simulink model "ASW_AST"  (R2023a)
settings: configuration reference "cfg_FastTaskCodeGeneration_v01" (kept outside this file)
undefined symbols (not defined in the file): Cdbl_tiSlwTaskSmpTi, Gu16_psiPermMagFlx_C
libraries: lib_conversion x1
settings Model: DataDictionary=dd_foc_dictionary.sldd  EnableAccessToBaseWorkspace=off  Creator=WFYXQ  LastModifiedBy=xiaoqiang.yuan
settings ConfigSetRef: SourceName=cfg_FastTaskCodeGeneration_v01

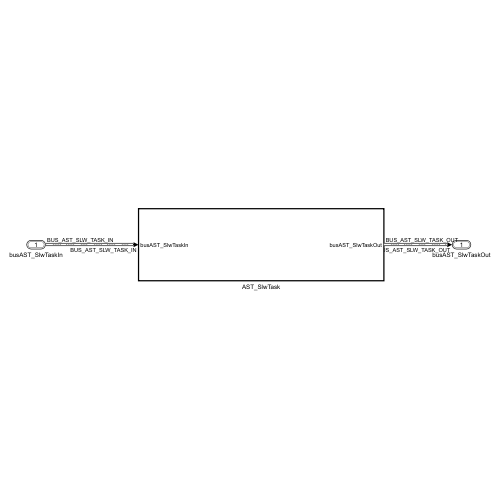
[thumbnail: Simulink's stored preview of the top-level diagram]
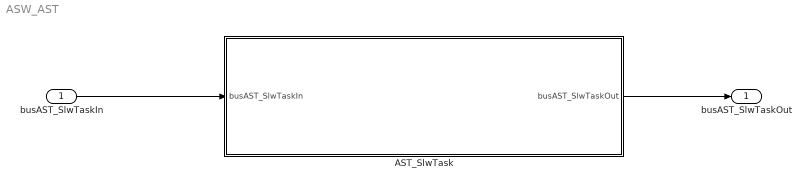
== system ASW_AST ==
  busAST_SlwTaskIn : Inport  OutDataTypeStr=Bus: BUS_AST_SLW_TASK_IN  SampleTime=round(double(Cdbl_tiSlwTaskSmpTi),4)  BusOutputAsStruct=on
  AST_SlwTask : Subsystem  TreatAsAtomicUnit=on  RTWFcnName=AST_SlwTask
      settings: RTWSystemCode=Nonreusable function  RTWFcnNameOpts=User specified
  busAST_SlwTaskOut : Outport  OutDataTypeStr=Bus: BUS_AST_SLW_TASK_OUT  SampleTime=round(double(Cdbl_tiSlwTaskSmpTi),4)
  wires:
  busAST_SlwTaskIn/1 -> AST_SlwTask/1(busAST_SlwTaskIn)
  AST_SlwTask/1(busAST_SlwTaskOut) -> busAST_SlwTaskOut/1

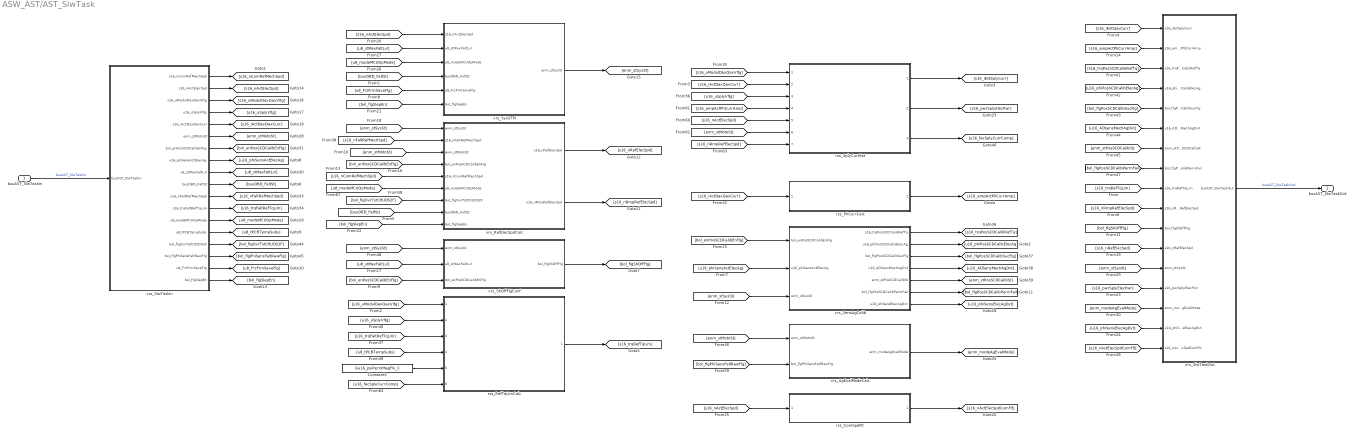
== system ASW_AST/AST_SlwTask ==
  busAST_SlwTaskIn : Inport
  Constant3 : Constant  Value=Gu16_psiPermMagFlx_C
  rss_ComSpdFlt : Subsystem  ReferencedSubsystem=rss_ComSpdFlt
  rss_PhCurrCalc : Subsystem  ReferencedSubsystem=rss_PhCurrCalc
  rss_RefTqLimCalc : Subsystem  ReferencedSubsystem=rss_RefTqLimCalc
  rss_SplyCurrEst : Subsystem  ReferencedSubsystem=rss_SplyCurrEst
  vrs_AgEvalModeCalc : Subsystem  Variant=on  VariantControlMode=label  VariantControl=Choice  LabelModeActiveChoice=cstHybrCtrlLbl
  vrs_RefElecSpdCalc : Subsystem  Variant=on  VariantControlMode=label  VariantControl=Choice  LabelModeActiveChoice=cstHybrCtrlLbl
  vrs_SensAgCalib : Subsystem  Variant=on  VariantControlMode=label  VariantControl=Choice  LabelModeActiveChoice=cstSensCtrlLbl
  vrs_ShOffFlgConf : Subsystem  Variant=on  VariantControlMode=label  VariantControl=Choice  LabelModeActiveChoice=cstSensCtrlLbl
  vrs_SlwTaskIn : Subsystem  Variant=on  VariantControlMode=label  VariantControl=cstSenlCtrlLbl  LabelModeActiveChoice=cstHybrCtrlLbl
  vrs_SlwTaskOut : Subsystem  Variant=on  VariantControlMode=label  VariantControl=Choice  LabelModeActiveChoice=cstHybrCtrlLbl
  vrs_SysSTM : Subsystem  Variant=on  VariantControlMode=label  VariantControl=Choice  LabelModeActiveChoice=GEELY_PROJECT
  busAST_SlwTaskOut : Outport
  wires:
  vrs_SensAgCalib/6(bol_flgPosSCDCalibPermFail) -> [bol_flgPosSCDCalibPermFail]
  vrs_SensAgCalib/5(enm_stPosSCDCalibSt) -> [enm_stPosSCDCalibSt]
  vrs_SensAgCalib/4(u16_ADSensMechAgDvt) -> [u16_ADSensMechAgDvt]
  vrs_SensAgCalib/2(u16_phiPosSCDCalibElecAg) -> [u16_phiPosSCDCalibElecAg]
  vrs_SensAgCalib/3(bol_flgPosSCDCalibSucFlg) -> [bol_flgPosSCDCalibSucFlg]
  [s16_iActDaxQaxCurr] -> rss_PhCurrCalc/1
  vrs_SlwTaskOut/1(busAST_SlwTaskOut) -> busAST_SlwTaskOut/1  "busAST_SlwTaskOut"
  [s16_iEstSplyCurr] -> vrs_SlwTaskOut/1(s16_iEstSplyCurr)
  [u16_uSplyVltg] -> rss_RefTqLimCalc/2
  [s16_uModulDaxQaxVltg] -> rss_SplyCurrEst/1
  rss_RefTqLimCalc/1 -> [s16_trqRefTqLim]
  rss_PhCurrCalc/1 -> [s16_ampActPhCurrAmp]
  [u16_uSplyVltg] -> rss_SplyCurrEst/3
  [s16_ampActPhCurrAmp] -> vrs_SlwTaskOut/2(s16_ampActPhCurrAmp)
  [bol_enPosSCDCalibEnFlg] -> vrs_SensAgCalib/1(bol_enPosSCDCalibEnFlg)
  [s16_iActDaxQaxCurr] -> rss_SplyCurrEst/2
  [s16_uModulDaxQaxVltg] -> rss_RefTqLimCalc/1
  [u16_phiPosSCDCalibElecAg] -> vrs_SlwTaskOut/4(u16_phiPosSCDCalibElecAg)
  [bol_flgPosSCDCalibPermFail] -> vrs_SlwTaskOut/8(bol_flgPosSCDCalibPermFail)
  [enm_stPosSCDCalibSt] -> vrs_SlwTaskOut/7(enm_stPosSCDCalibSt)
  [u16_ADSensMechAgDvt] -> vrs_SlwTaskOut/6(u16_ADSensMechAgDvt)
  [bol_flgPosSCDCalibSucFlg] -> vrs_SlwTaskOut/5(bol_flgPosSCDCalibSucFlg)
  [s16_trqPosSCDCalibRefTq] -> vrs_SlwTaskOut/3(s16_trqPosSCDCalibRefTq)
  vrs_SensAgCalib/1(s16_trqPosSCDCalibRefTq) -> [s16_trqPosSCDCalibRefTq]
  rss_SplyCurrEst/1 -> [s16_iEstSplyCurr]
  [s16_trqRefTqLim] -> vrs_SlwTaskOut/9(s16_trqRefTqLim)
  [s16_nRmpRefElecSpd] -> vrs_SlwTaskOut/10(s16_nRmpRefElecSpd)
  [bol_flgShOffFlg] -> vrs_SlwTaskOut/11(bol_flgShOffFlg)
  [u16_phiSensActElecAg] -> vrs_SensAgCalib/2(u16_phiSensActElecAg)
  [s16_nRefElecSpd] -> vrs_SlwTaskOut/12(s16_nRefElecSpd)
  [enm_stSysSt] -> vrs_SlwTaskOut/13(enm_stSysSt)
  [s16_trqFaltRefTqLim] -> rss_RefTqLimCalc/3
  [u8_tPCBTempSubs] -> rss_RefTqLimCalc/4
  [enm_stSysSt] -> vrs_SensAgCalib/3(enm_stSysSt)
  Constant3/1 -> rss_RefTqLimCalc/5
  [enm_stSysSt] -> vrs_ShOffFlgConf/1(enm_stSysSt)
  [u8_stMaxFaltLvl] -> vrs_ShOffFlgConf/2(u8_stMaxFaltLvl)
  [bol_enPosSCDCalibEnFlg] -> vrs_ShOffFlgConf/3(bol_enPosSCDCalibEnFlg)
  vrs_ShOffFlgConf/1(bol_flgShOffFlg) -> [bol_flgShOffFlg]
  [enm_stSysSt] -> vrs_RefElecSpdCalc/1(enm_stSysSt)
  [s16_nFaltRefMechSpd] -> vrs_RefElecSpdCalc/2(s16_nFaltRefMechSpd)
  [enm_stMotoSt] -> vrs_RefElecSpdCalc/3(enm_stMotoSt)
  [bol_enPosSCDCalibEnFlg] -> vrs_RefElecSpdCalc/4(bol_enPosSCDCalibEnFlg)
  [s16_nComRefMechSpd] -> vrs_RefElecSpdCalc/5(s16_nComRefMechSpd)
  vrs_RefElecSpdCalc/1(s16_nRefElecSpd) -> [s16_nRefElecSpd]
  vrs_RefElecSpdCalc/2(s16_nRmpRefElecSpd) -> [s16_nRmpRefElecSpd]
  [u8_modeMCUOpMode] -> vrs_RefElecSpdCalc/6(u8_modeMCUOpMode)
  rss_SplyCurrEst/2 -> [s16_pwrSplyElecPwr]
  [s16_pwrSplyElecPwr] -> vrs_SlwTaskOut/14(s16_pwrSplyElecPwr)
  [bol_flgOvrTstCtlUDS2F] -> vrs_RefElecSpdCalc/7(bol_flgOvrTstCtlUDS2F)
  [enm_modeAgEvalMode] -> vrs_SlwTaskOut/15(enm_modeAgEvalMode)
  busAST_SlwTaskIn/1 -> vrs_SlwTaskIn/1(busAST_SlwTaskIn)  "busAST_SlwTaskIn"
  vrs_SlwTaskIn/1(s16_nComRefMechSpd) -> [s16_nComRefMechSpd]
  vrs_SlwTaskIn/2(s16_nActElecSpd) -> [s16_nActElecSpd]
  vrs_SlwTaskIn/3(s16_uModulDaxQaxVltg) -> [s16_uModulDaxQaxVltg]
  vrs_SlwTaskIn/4(u16_uSplyVltg) -> [u16_uSplyVltg]
  vrs_SlwTaskIn/5(s16_iActDaxQaxCurr) -> [s16_iActDaxQaxCurr]
  vrs_SlwTaskIn/6(enm_stMotoSt) -> [enm_stMotoSt]
  vrs_SlwTaskIn/7(bol_enPosSCDCalibEnFlg) -> [bol_enPosSCDCalibEnFlg]
  vrs_SlwTaskIn/8(u16_phiSensActElecAg) -> [u16_phiSensActElecAg]
  vrs_SlwTaskIn/9(u8_stMaxFaltLvl) -> [u8_stMaxFaltLvl]
  vrs_SlwTaskIn/10(busOBD_FaltSt) -> [busOBD_FaltSt]
  vrs_SlwTaskIn/11(s16_nFaltRefMechSpd) -> [s16_nFaltRefMechSpd]
  vrs_SlwTaskIn/12(s16_trqFaltRefTqLim) -> [s16_trqFaltRefTqLim]
  vrs_SlwTaskIn/13(u8_modeMCUOpMode) -> [u8_modeMCUOpMode]
  vrs_SlwTaskIn/14(u8_tPCBTempSubs) -> [u8_tPCBTempSubs]
  vrs_SlwTaskIn/15(bol_flgOvrTstCtlUDS2F) -> [bol_flgOvrTstCtlUDS2F]
  vrs_AgEvalModeCalc/1(enm_modeAgEvalMode) -> [enm_modeAgEvalMode]
  [enm_stMotoSt] -> vrs_AgEvalModeCalc/1(enm_stMotoSt)
  [bol_flgPhiSensFaltRawFlg] -> vrs_AgEvalModeCalc/2(bol_flgPhiSensFaltRawFlg)
  vrs_SlwTaskIn/16(bol_flgPhiSensFaltRawFlg) -> [bol_flgPhiSensFaltRawFlg]
  [s16_ampActPhCurrAmp] -> rss_SplyCurrEst/4
  [s16_nActElecSpd] -> rss_SplyCurrEst/5
  [enm_stMotoSt] -> rss_SplyCurrEst/6
  [s16_nRmpRefElecSpd] -> rss_SplyCurrEst/7
  rss_SplyCurrEst/3 -> [u16_facSplyCurrComp]
  [u16_facSplyCurrComp] -> rss_RefTqLimCalc/6
  [busOBD_FaltSt] -> vrs_RefElecSpdCalc/8(busOBD_FaltSt)
  vrs_SlwTaskIn/17(u8_FrzFrmSaveFlg) -> [u8_FrzFrmSaveFlg]
  [s16_nActElecSpd] -> vrs_SysSTM/1(s16_nActElecSpd)
  [u8_stMaxFaltLvl] -> vrs_SysSTM/2(u8_stMaxFaltLvl)
  [u8_modeMCUOpMode] -> vrs_SysSTM/3(u8_modeMCUOpMode)
  [busOBD_FaltSt] -> vrs_SysSTM/4(busOBD_FaltSt)
  [u8_FrzFrmSaveFlg] -> vrs_SysSTM/5(u8_FrzFrmSaveFlg)
  vrs_SysSTM/1(enm_stSysSt) -> [enm_stSysSt]
  [bol_flgSlepEn] -> vrs_SysSTM/6(bol_flgSlepEn)
  [bol_flgSlepEn] -> vrs_RefElecSpdCalc/9(bol_flgSlepEn)
  vrs_SlwTaskIn/18(bol_flgSlepEn) -> [bol_flgSlepEn]
  vrs_SensAgCalib/7(u16_phiSensElecAgDvt) -> [u16_phiSensElecAgDvt]
  [u16_phiSensElecAgDvt] -> vrs_SlwTaskOut/16(u16_phiSensElecAgDvt)
  [s16_nActElecSpd] -> rss_ComSpdFlt/1
  rss_ComSpdFlt/1 -> [s16_nActElecSpdComFlt]
  [s16_nActElecSpdComFlt] -> vrs_SlwTaskOut/17(s16_nActElecSpdComFlt)

== system ASW_AST/AST_SlwTask/vrs_AgEvalModeCalc ==
  enm_stMotoSt : Inport
  bol_flgPhiSensFaltRawFlg : Inport  Port=2
  rss_AgEvalModeCalcNeed : Subsystem  VariantControl=cstHybrCtrlLbl  ReferencedSubsystem=rss_AgEvalModeCalcNeed
  rss_AgEvalModeCalcNoNeed : Subsystem  VariantControl=cstSensCtrlLbl
  enm_modeAgEvalMode : Outport

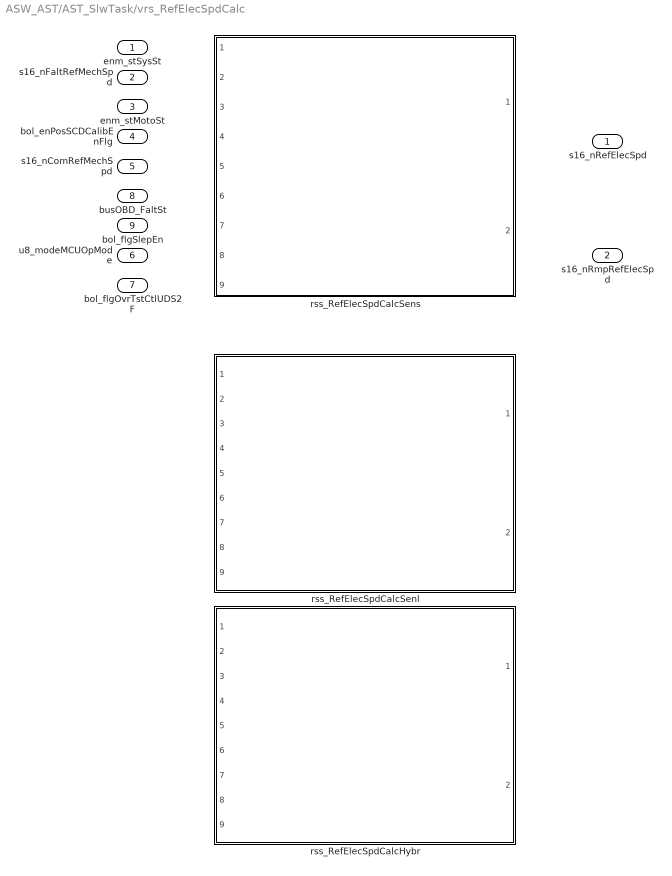
== system ASW_AST/AST_SlwTask/vrs_RefElecSpdCalc ==
  enm_stSysSt : Inport
  s16_nFaltRefMechSpd : Inport  Port=2
  enm_stMotoSt : Inport  Port=3
  bol_enPosSCDCalibEnFlg : Inport  Port=4
  s16_nComRefMechSpd : Inport  Port=5
  u8_modeMCUOpMode : Inport  Port=6
  bol_flgOvrTstCtlUDS2F : Inport  Port=7  OutDataTypeStr=boolean
  busOBD_FaltSt : Inport  Port=8  OutDataTypeStr=Bus: BUS_OBD_FALT_STS
  bol_flgSlepEn : Inport  Port=9
  rss_RefElecSpdCalcHybr : Subsystem  VariantControl=cstHybrCtrlLbl  ReferencedSubsystem=rss_RefElecSpdCalcHybr
  rss_RefElecSpdCalcSenl : Subsystem  VariantControl=cstSenlCtrlLbl  ReferencedSubsystem=rss_RefElecSpdCalcSenl
  rss_RefElecSpdCalcSens : Subsystem  VariantControl=cstSensCtrlLbl  ReferencedSubsystem=rss_RefElecSpdCalcSens
  s16_nRefElecSpd : Outport
  s16_nRmpRefElecSpd : Outport  Port=2

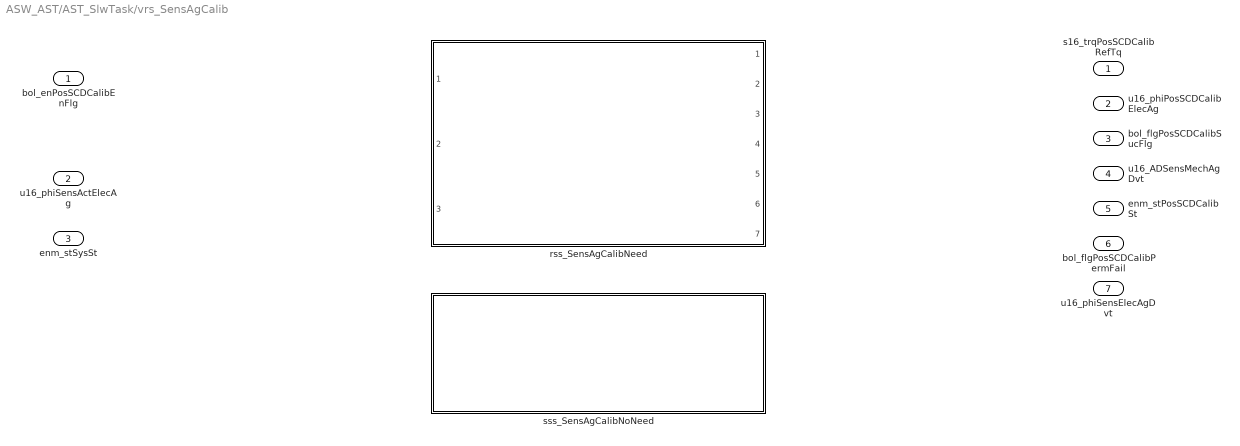
== system ASW_AST/AST_SlwTask/vrs_SensAgCalib ==
  bol_enPosSCDCalibEnFlg : Inport
  u16_phiSensActElecAg : Inport  Port=2
  enm_stSysSt : Inport  Port=3
  rss_SensAgCalibNeed : Subsystem  VariantControl=cstSensCtrlLbl  ReferencedSubsystem=rss_SensAgCalibNeed
  sss_SensAgCalibNoNeed : Subsystem  VariantControl=cstSenlCtrlLbl
  s16_trqPosSCDCalibRefTq : Outport
  u16_phiPosSCDCalibElecAg : Outport  Port=2
  bol_flgPosSCDCalibSucFlg : Outport  Port=3
  u16_ADSensMechAgDvt : Outport  Port=4
  enm_stPosSCDCalibSt : Outport  Port=5
  bol_flgPosSCDCalibPermFail : Outport  Port=6
  u16_phiSensElecAgDvt : Outport  Port=7

== system ASW_AST/AST_SlwTask/vrs_ShOffFlgConf ==
  enm_stSysSt : Inport
  u8_stMaxFaltLvl : Inport  Port=2
  bol_enPosSCDCalibEnFlg : Inport  Port=3
  rss_ShOffFlgConfSenl : Subsystem  VariantControl=cstSenlCtrlLbl  ReferencedSubsystem=rss_ShOffFlgConfSenl
  rss_ShOffFlgConfSens : Subsystem  VariantControl=cstSensCtrlLbl  ReferencedSubsystem=rss_ShOffFlgConfSens
  bol_flgShOffFlg : Outport

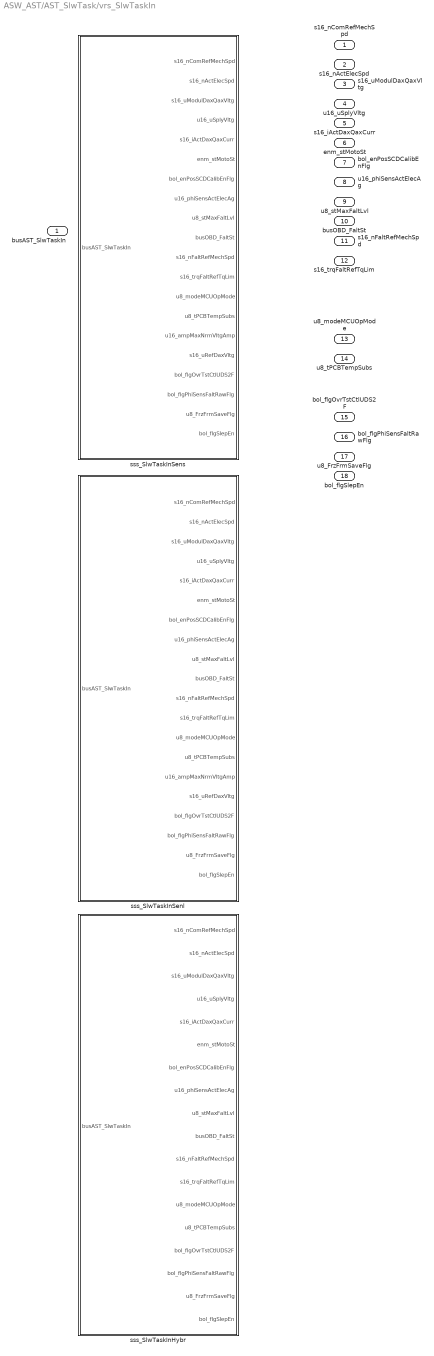
== system ASW_AST/AST_SlwTask/vrs_SlwTaskIn ==
  busAST_SlwTaskIn : Inport
  sss_SlwTaskInHybr : Subsystem  VariantControl=cstHybrCtrlLbl
  sss_SlwTaskInSenl : Subsystem  VariantControl=cstSenlCtrlLbl
  sss_SlwTaskInSens : Subsystem  VariantControl=cstSensCtrlLbl
  s16_nComRefMechSpd : Outport
  s16_nActElecSpd : Outport  Port=2
  s16_uModulDaxQaxVltg : Outport  Port=3
  u16_uSplyVltg : Outport  Port=4
  s16_iActDaxQaxCurr : Outport  Port=5
  enm_stMotoSt : Outport  Port=6
  bol_enPosSCDCalibEnFlg : Outport  Port=7
  u16_phiSensActElecAg : Outport  Port=8
  u8_stMaxFaltLvl : Outport  Port=9
  busOBD_FaltSt : Outport  Port=10
  s16_nFaltRefMechSpd : Outport  Port=11
  s16_trqFaltRefTqLim : Outport  Port=12
  u8_modeMCUOpMode : Outport  Port=13
  u8_tPCBTempSubs : Outport  Port=14
  bol_flgOvrTstCtlUDS2F : Outport  Port=15
  bol_flgPhiSensFaltRawFlg : Outport  Port=16
  u8_FrzFrmSaveFlg : Outport  Port=17
  bol_flgSlepEn : Outport  Port=18

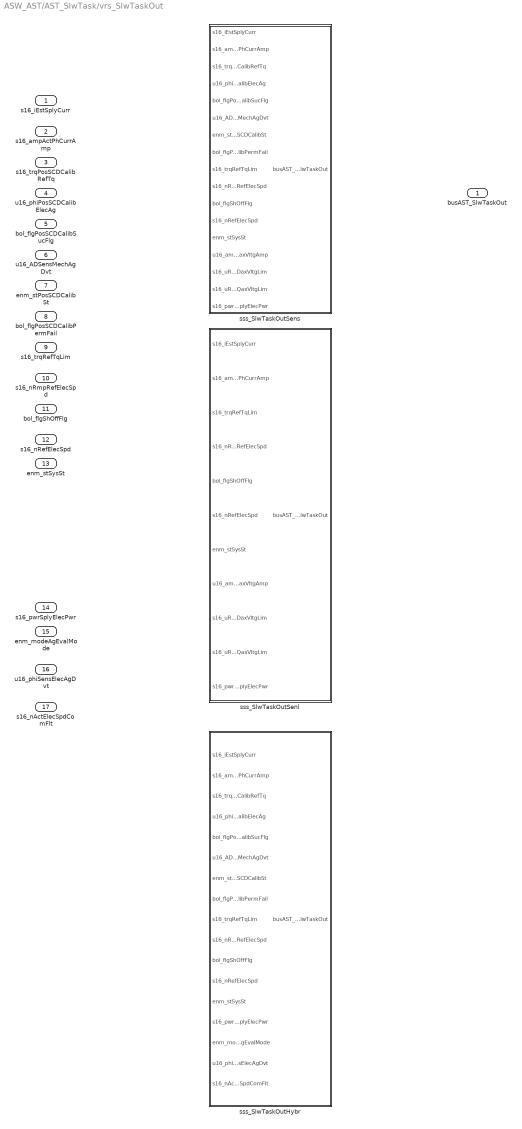
== system ASW_AST/AST_SlwTask/vrs_SlwTaskOut ==
  s16_iEstSplyCurr : Inport
  s16_ampActPhCurrAmp : Inport  Port=2
  s16_trqPosSCDCalibRefTq : Inport  Port=3
  u16_phiPosSCDCalibElecAg : Inport  Port=4
  bol_flgPosSCDCalibSucFlg : Inport  Port=5
  u16_ADSensMechAgDvt : Inport  Port=6
  enm_stPosSCDCalibSt : Inport  Port=7
  bol_flgPosSCDCalibPermFail : Inport  Port=8
  s16_trqRefTqLim : Inport  Port=9
  s16_nRmpRefElecSpd : Inport  Port=10
  bol_flgShOffFlg : Inport  Port=11
  s16_nRefElecSpd : Inport  Port=12
  enm_stSysSt : Inport  Port=13
  s16_pwrSplyElecPwr : Inport  Port=14
  enm_modeAgEvalMode : Inport  Port=15
  u16_phiSensElecAgDvt : Inport  Port=16
  s16_nActElecSpdComFlt : Inport  Port=17
  sss_SlwTaskOutHybr : Subsystem  VariantControl=cstHybrCtrlLbl
  sss_SlwTaskOutSenl : Subsystem  VariantControl=cstSenlCtrlLbl
  sss_SlwTaskOutSens : Subsystem  VariantControl=cstSensCtrlLbl
  busAST_SlwTaskOut : Outport

== system ASW_AST/AST_SlwTask/vrs_SysSTM ==
  s16_nActElecSpd : Inport
  u8_stMaxFaltLvl : Inport  Port=2
  u8_modeMCUOpMode : Inport  Port=3
  busOBD_FaltSt : Inport  Port=4
  u8_FrzFrmSaveFlg : Inport  Port=5
  bol_flgSlepEn : Inport  Port=6
  rss_SysSTM_CRRC : Subsystem  VariantControl=CRRC_PROJECT  ReferencedSubsystem=rss_SysSTM_CRRC
  rss_SysSTM_GEELY : Subsystem  VariantControl=GEELY_PROJECT  ReferencedSubsystem=rss_SysSTM_GEELY
  enm_stSysSt : Outport

== system ASW_AST/AST_SlwTask/vrs_AgEvalModeCalc/rss_AgEvalModeCalcNoNeed ==
  enm_stMotoSt : Inport  OutDataTypeStr=Enum: ENM_MOTO_STATUS
  bol_flgPhiSensFaltRawFlg : Inport  Port=2  OutDataTypeStr=boolean
  Ground : Ground
  Terminator : Terminator
  Terminator1 : Terminator
  lib_Cnvr_3 : lib_conversion/lib_Conversion_0  lb_parDataType=Inherit: Inherit via back propagation  lb_parOutpMaxVal=[]  lb_parOutpMinVal=[]  lb_parSatFlag=off
  enm_modeAgEvalMode : Outport
  wires:
  enm_stMotoSt/1 -> Terminator/1
  bol_flgPhiSensFaltRawFlg/1 -> Terminator1/1
  Ground/1 -> lib_Cnvr_3/1
  lib_Cnvr_3/1 -> enm_modeAgEvalMode/1

== system ASW_AST/AST_SlwTask/vrs_SensAgCalib/sss_SensAgCalibNoNeed ==

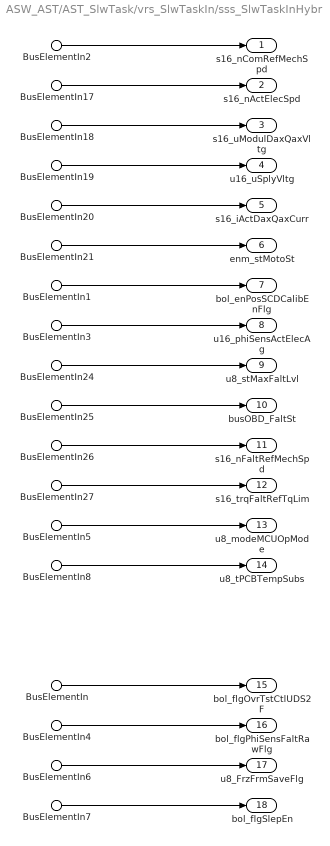
== system ASW_AST/AST_SlwTask/vrs_SlwTaskIn/sss_SlwTaskInHybr ==
  BusElementIn2 : Inport  PortName=busAST_SlwTaskIn  Element=s16_nComRefMechSpd
  BusElementIn17 : Inport  PortName=busAST_SlwTaskIn  Element=s16_nActElecSpd
  BusElementIn18 : Inport  PortName=busAST_SlwTaskIn  Element=s16_uModulDaxQaxVltg
  BusElementIn19 : Inport  PortName=busAST_SlwTaskIn  Element=u16_uSplyVltg
  BusElementIn20 : Inport  PortName=busAST_SlwTaskIn  Element=s16_iActDaxQaxCurr
  BusElementIn21 : Inport  PortName=busAST_SlwTaskIn  Element=enm_stMotoSt
  BusElementIn24 : Inport  PortName=busAST_SlwTaskIn  Element=u8_stMaxFaltLvl
  BusElementIn25 : Inport  PortName=busAST_SlwTaskIn  Element=busOBD_FaltSt
  BusElementIn26 : Inport  PortName=busAST_SlwTaskIn  Element=s16_nFaltRefMechSpd
  BusElementIn27 : Inport  PortName=busAST_SlwTaskIn  Element=s16_trqFaltRefTqLim
  BusElementIn : Inport  PortName=busAST_SlwTaskIn  Element=bol_flgOvrTstCtlUDS2F
  BusElementIn1 : Inport  PortName=busAST_SlwTaskIn  Element=bol_enPosSCDCalibEnFlg
  BusElementIn3 : Inport  PortName=busAST_SlwTaskIn  Element=u16_phiSensActElecAg
  BusElementIn4 : Inport  PortName=busAST_SlwTaskIn  Element=bol_flgPhiSensFaltRawFlg
  BusElementIn5 : Inport  PortName=busAST_SlwTaskIn  Element=u8_modeMCUOpMode
  BusElementIn6 : Inport  PortName=busAST_SlwTaskIn  Element=u8_FrzFrmSaveFlg
  BusElementIn7 : Inport  PortName=busAST_SlwTaskIn  Element=bol_flgSlepEn
  BusElementIn8 : Inport  PortName=busAST_SlwTaskIn  Element=u8_tPCBTempSubs
  s16_nComRefMechSpd : Outport
  s16_nActElecSpd : Outport  Port=2
  s16_uModulDaxQaxVltg : Outport  Port=3
  u16_uSplyVltg : Outport  Port=4
  s16_iActDaxQaxCurr : Outport  Port=5
  enm_stMotoSt : Outport  Port=6
  bol_enPosSCDCalibEnFlg : Outport  Port=7
  u16_phiSensActElecAg : Outport  Port=8
  u8_stMaxFaltLvl : Outport  Port=9
  busOBD_FaltSt : Outport  Port=10
  s16_nFaltRefMechSpd : Outport  Port=11
  s16_trqFaltRefTqLim : Outport  Port=12
  u8_modeMCUOpMode : Outport  Port=13
  u8_tPCBTempSubs : Outport  Port=14
  bol_flgOvrTstCtlUDS2F : Outport  Port=15
  bol_flgPhiSensFaltRawFlg : Outport  Port=16
  u8_FrzFrmSaveFlg : Outport  Port=17
  bol_flgSlepEn : Outport  Port=18
  wires:
  BusElementIn/1 -> bol_flgOvrTstCtlUDS2F/1
  BusElementIn21/1 -> enm_stMotoSt/1
  BusElementIn24/1 -> u8_stMaxFaltLvl/1
  BusElementIn25/1 -> busOBD_FaltSt/1
  BusElementIn26/1 -> s16_nFaltRefMechSpd/1
  BusElementIn27/1 -> s16_trqFaltRefTqLim/1
  BusElementIn5/1 -> u8_modeMCUOpMode/1
  BusElementIn8/1 -> u8_tPCBTempSubs/1
  BusElementIn20/1 -> s16_iActDaxQaxCurr/1
  BusElementIn19/1 -> u16_uSplyVltg/1
  BusElementIn18/1 -> s16_uModulDaxQaxVltg/1
  BusElementIn17/1 -> s16_nActElecSpd/1
  BusElementIn2/1 -> s16_nComRefMechSpd/1
  BusElementIn1/1 -> bol_enPosSCDCalibEnFlg/1
  BusElementIn3/1 -> u16_phiSensActElecAg/1
  BusElementIn4/1 -> bol_flgPhiSensFaltRawFlg/1
  BusElementIn6/1 -> u8_FrzFrmSaveFlg/1
  BusElementIn7/1 -> bol_flgSlepEn/1

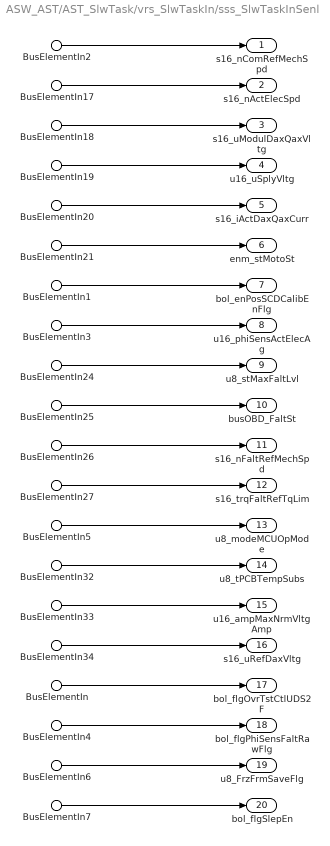
== system ASW_AST/AST_SlwTask/vrs_SlwTaskIn/sss_SlwTaskInSenl ==
  BusElementIn2 : Inport  PortName=busAST_SlwTaskIn  Element=s16_nComRefMechSpd
  BusElementIn17 : Inport  PortName=busAST_SlwTaskIn  Element=s16_nActElecSpd
  BusElementIn18 : Inport  PortName=busAST_SlwTaskIn  Element=s16_uModulDaxQaxVltg
  BusElementIn19 : Inport  PortName=busAST_SlwTaskIn  Element=u16_uSplyVltg
  BusElementIn20 : Inport  PortName=busAST_SlwTaskIn  Element=s16_iActDaxQaxCurr
  BusElementIn21 : Inport  PortName=busAST_SlwTaskIn  Element=enm_stMotoSt
  BusElementIn24 : Inport  PortName=busAST_SlwTaskIn  Element=u8_stMaxFaltLvl
  BusElementIn25 : Inport  PortName=busAST_SlwTaskIn  Element=busOBD_FaltSt
  BusElementIn26 : Inport  PortName=busAST_SlwTaskIn  Element=s16_nFaltRefMechSpd
  BusElementIn27 : Inport  PortName=busAST_SlwTaskIn  Element=s16_trqFaltRefTqLim
  BusElementIn32 : Inport  PortName=busAST_SlwTaskIn  Element=u8_tPCBTemp
  BusElementIn33 : Inport  PortName=busAST_SlwTaskIn  Element=u16_ampMaxNrmVltgAmp
  BusElementIn34 : Inport  PortName=busAST_SlwTaskIn  Element=s16_uRefDaxVltg
  BusElementIn : Inport  PortName=busAST_SlwTaskIn  Element=bol_flgOvrTstCtlUDS2F
  BusElementIn1 : Inport  PortName=busAST_SlwTaskIn  Element=bol_enPosSCDCalibEnFlg
  BusElementIn3 : Inport  PortName=busAST_SlwTaskIn  Element=u16_phiSensActElecAg
  BusElementIn4 : Inport  PortName=busAST_SlwTaskIn  Element=bol_flgPhiSensFaltRawFlg
  BusElementIn5 : Inport  PortName=busAST_SlwTaskIn  Element=u8_modeMCUOpMode
  BusElementIn6 : Inport  PortName=busAST_SlwTaskIn  Element=u8_FrzFrmSaveFlg
  BusElementIn7 : Inport  PortName=busAST_SlwTaskIn  Element=bol_flgSlepEn
  s16_nComRefMechSpd : Outport
  s16_nActElecSpd : Outport  Port=2
  s16_uModulDaxQaxVltg : Outport  Port=3
  u16_uSplyVltg : Outport  Port=4
  s16_iActDaxQaxCurr : Outport  Port=5
  enm_stMotoSt : Outport  Port=6
  bol_enPosSCDCalibEnFlg : Outport  Port=7
  u16_phiSensActElecAg : Outport  Port=8
  u8_stMaxFaltLvl : Outport  Port=9
  busOBD_FaltSt : Outport  Port=10
  s16_nFaltRefMechSpd : Outport  Port=11
  s16_trqFaltRefTqLim : Outport  Port=12
  u8_modeMCUOpMode : Outport  Port=13
  u8_tPCBTempSubs : Outport  Port=14
  u16_ampMaxNrmVltgAmp : Outport  Port=15
  s16_uRefDaxVltg : Outport  Port=16
  bol_flgOvrTstCtlUDS2F : Outport  Port=17
  bol_flgPhiSensFaltRawFlg : Outport  Port=18
  u8_FrzFrmSaveFlg : Outport  Port=19
  bol_flgSlepEn : Outport  Port=20
  wires:
  BusElementIn17/1 -> s16_nActElecSpd/1
  BusElementIn7/1 -> bol_flgSlepEn/1
  BusElementIn2/1 -> s16_nComRefMechSpd/1
  BusElementIn18/1 -> s16_uModulDaxQaxVltg/1
  BusElementIn3/1 -> u16_phiSensActElecAg/1
  BusElementIn1/1 -> bol_enPosSCDCalibEnFlg/1
  BusElementIn6/1 -> u8_FrzFrmSaveFlg/1
  BusElementIn/1 -> bol_flgOvrTstCtlUDS2F/1
  BusElementIn34/1 -> s16_uRefDaxVltg/1
  BusElementIn4/1 -> bol_flgPhiSensFaltRawFlg/1
  BusElementIn20/1 -> s16_iActDaxQaxCurr/1
  BusElementIn19/1 -> u16_uSplyVltg/1
  BusElementIn24/1 -> u8_stMaxFaltLvl/1
  BusElementIn32/1 -> u8_tPCBTempSubs/1
  BusElementIn27/1 -> s16_trqFaltRefTqLim/1
  BusElementIn25/1 -> busOBD_FaltSt/1
  BusElementIn26/1 -> s16_nFaltRefMechSpd/1
  BusElementIn21/1 -> enm_stMotoSt/1
  BusElementIn5/1 -> u8_modeMCUOpMode/1
  BusElementIn33/1 -> u16_ampMaxNrmVltgAmp/1

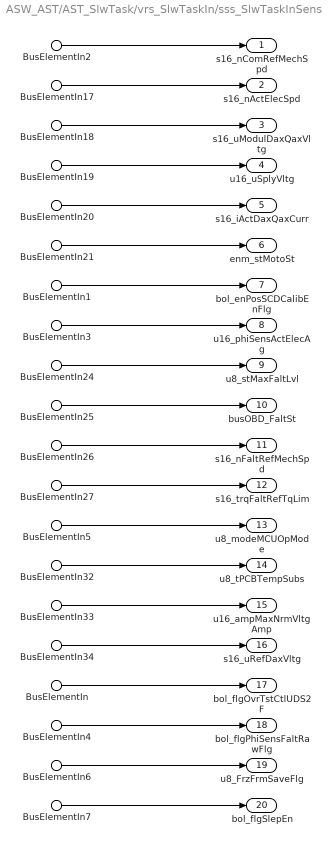
== system ASW_AST/AST_SlwTask/vrs_SlwTaskIn/sss_SlwTaskInSens ==
  BusElementIn2 : Inport  PortName=busAST_SlwTaskIn  Element=s16_nComRefMechSpd
  BusElementIn17 : Inport  PortName=busAST_SlwTaskIn  Element=s16_nActElecSpd
  BusElementIn18 : Inport  PortName=busAST_SlwTaskIn  Element=s16_uModulDaxQaxVltg
  BusElementIn19 : Inport  PortName=busAST_SlwTaskIn  Element=u16_uSplyVltg
  BusElementIn20 : Inport  PortName=busAST_SlwTaskIn  Element=s16_iActDaxQaxCurr
  BusElementIn21 : Inport  PortName=busAST_SlwTaskIn  Element=enm_stMotoSt
  BusElementIn24 : Inport  PortName=busAST_SlwTaskIn  Element=u8_stMaxFaltLvl
  BusElementIn25 : Inport  PortName=busAST_SlwTaskIn  Element=busOBD_FaltSt
  BusElementIn26 : Inport  PortName=busAST_SlwTaskIn  Element=s16_nFaltRefMechSpd
  BusElementIn27 : Inport  PortName=busAST_SlwTaskIn  Element=s16_trqFaltRefTqLim
  BusElementIn32 : Inport  PortName=busAST_SlwTaskIn  Element=u8_tPCBTemp
  BusElementIn33 : Inport  PortName=busAST_SlwTaskIn  Element=u16_ampMaxNrmVltgAmp
  BusElementIn34 : Inport  PortName=busAST_SlwTaskIn  Element=s16_uRefDaxVltg
  BusElementIn : Inport  PortName=busAST_SlwTaskIn  Element=bol_flgOvrTstCtlUDS2F
  BusElementIn1 : Inport  PortName=busAST_SlwTaskIn  Element=bol_enPosSCDCalibEnFlg
  BusElementIn3 : Inport  PortName=busAST_SlwTaskIn  Element=u16_phiSensActElecAg
  BusElementIn4 : Inport  PortName=busAST_SlwTaskIn  Element=bol_flgPhiSensFaltRawFlg
  BusElementIn5 : Inport  PortName=busAST_SlwTaskIn  Element=u8_modeMCUOpMode
  BusElementIn6 : Inport  PortName=busAST_SlwTaskIn  Element=u8_FrzFrmSaveFlg
  BusElementIn7 : Inport  PortName=busAST_SlwTaskIn  Element=bol_flgSlepEn
  s16_nComRefMechSpd : Outport
  s16_nActElecSpd : Outport  Port=2
  s16_uModulDaxQaxVltg : Outport  Port=3
  u16_uSplyVltg : Outport  Port=4
  s16_iActDaxQaxCurr : Outport  Port=5
  enm_stMotoSt : Outport  Port=6
  bol_enPosSCDCalibEnFlg : Outport  Port=7
  u16_phiSensActElecAg : Outport  Port=8
  u8_stMaxFaltLvl : Outport  Port=9
  busOBD_FaltSt : Outport  Port=10
  s16_nFaltRefMechSpd : Outport  Port=11
  s16_trqFaltRefTqLim : Outport  Port=12
  u8_modeMCUOpMode : Outport  Port=13
  u8_tPCBTempSubs : Outport  Port=14
  u16_ampMaxNrmVltgAmp : Outport  Port=15
  s16_uRefDaxVltg : Outport  Port=16
  bol_flgOvrTstCtlUDS2F : Outport  Port=17
  bol_flgPhiSensFaltRawFlg : Outport  Port=18
  u8_FrzFrmSaveFlg : Outport  Port=19
  bol_flgSlepEn : Outport  Port=20
  wires:
  BusElementIn17/1 -> s16_nActElecSpd/1
  BusElementIn7/1 -> bol_flgSlepEn/1
  BusElementIn2/1 -> s16_nComRefMechSpd/1
  BusElementIn18/1 -> s16_uModulDaxQaxVltg/1
  BusElementIn3/1 -> u16_phiSensActElecAg/1
  BusElementIn1/1 -> bol_enPosSCDCalibEnFlg/1
  BusElementIn6/1 -> u8_FrzFrmSaveFlg/1
  BusElementIn/1 -> bol_flgOvrTstCtlUDS2F/1
  BusElementIn34/1 -> s16_uRefDaxVltg/1
  BusElementIn4/1 -> bol_flgPhiSensFaltRawFlg/1
  BusElementIn20/1 -> s16_iActDaxQaxCurr/1
  BusElementIn19/1 -> u16_uSplyVltg/1
  BusElementIn24/1 -> u8_stMaxFaltLvl/1
  BusElementIn32/1 -> u8_tPCBTempSubs/1
  BusElementIn27/1 -> s16_trqFaltRefTqLim/1
  BusElementIn25/1 -> busOBD_FaltSt/1
  BusElementIn26/1 -> s16_nFaltRefMechSpd/1
  BusElementIn21/1 -> enm_stMotoSt/1
  BusElementIn5/1 -> u8_modeMCUOpMode/1
  BusElementIn33/1 -> u16_ampMaxNrmVltgAmp/1

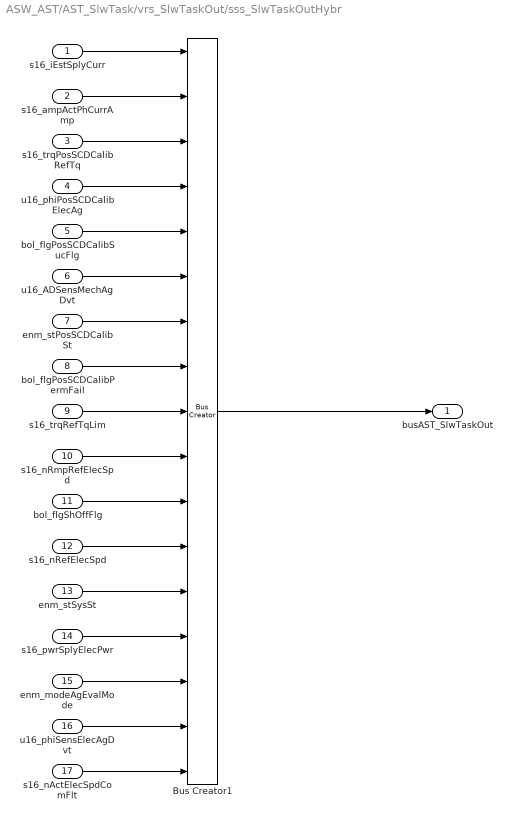
== system ASW_AST/AST_SlwTask/vrs_SlwTaskOut/sss_SlwTaskOutHybr ==
  s16_iEstSplyCurr : Inport
  s16_ampActPhCurrAmp : Inport  Port=2
  s16_trqPosSCDCalibRefTq : Inport  Port=3
  u16_phiPosSCDCalibElecAg : Inport  Port=4
  bol_flgPosSCDCalibSucFlg : Inport  Port=5
  u16_ADSensMechAgDvt : Inport  Port=6
  enm_stPosSCDCalibSt : Inport  Port=7
  bol_flgPosSCDCalibPermFail : Inport  Port=8
  s16_trqRefTqLim : Inport  Port=9
  s16_nRmpRefElecSpd : Inport  Port=10
  bol_flgShOffFlg : Inport  Port=11
  s16_nRefElecSpd : Inport  Port=12
  enm_stSysSt : Inport  Port=13
  s16_pwrSplyElecPwr : Inport  Port=14
  enm_modeAgEvalMode : Inport  Port=15
  u16_phiSensElecAgDvt : Inport  Port=16
  s16_nActElecSpdComFlt : Inport  Port=17
  Bus Creator1 : BusCreator  Inputs=17  OutDataTypeStr=Bus: BUS_AST_SLW_TASK_OUT  NonVirtualBus=on
      settings: InheritFromInputs=off
  busAST_SlwTaskOut : Outport
  wires:
  u16_phiPosSCDCalibElecAg/1 -> Bus Creator1/4
  bol_flgShOffFlg/1 -> Bus Creator1/11
  bol_flgPosSCDCalibSucFlg/1 -> Bus Creator1/5
  enm_stPosSCDCalibSt/1 -> Bus Creator1/7
  s16_ampActPhCurrAmp/1 -> Bus Creator1/2
  bol_flgPosSCDCalibPermFail/1 -> Bus Creator1/8
  s16_trqRefTqLim/1 -> Bus Creator1/9
  s16_trqPosSCDCalibRefTq/1 -> Bus Creator1/3
  s16_nRmpRefElecSpd/1 -> Bus Creator1/10
  Bus Creator1/1 -> busAST_SlwTaskOut/1
  u16_ADSensMechAgDvt/1 -> Bus Creator1/6
  s16_iEstSplyCurr/1 -> Bus Creator1/1
  s16_nRefElecSpd/1 -> Bus Creator1/12
  enm_stSysSt/1 -> Bus Creator1/13
  s16_pwrSplyElecPwr/1 -> Bus Creator1/14
  enm_modeAgEvalMode/1 -> Bus Creator1/15
  u16_phiSensElecAgDvt/1 -> Bus Creator1/16
  s16_nActElecSpdComFlt/1 -> Bus Creator1/17

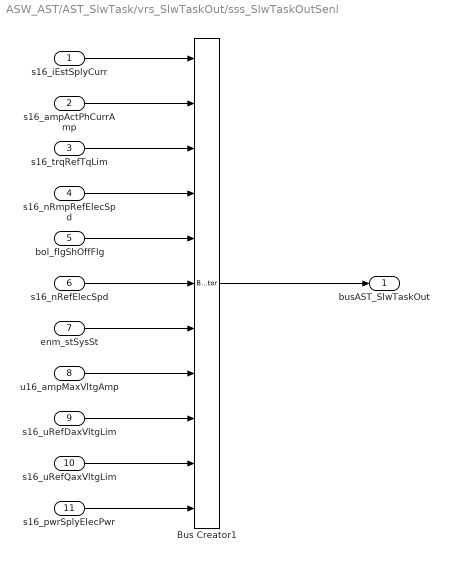
== system ASW_AST/AST_SlwTask/vrs_SlwTaskOut/sss_SlwTaskOutSenl ==
  s16_iEstSplyCurr : Inport
  s16_ampActPhCurrAmp : Inport  Port=2
  s16_trqRefTqLim : Inport  Port=3
  s16_nRmpRefElecSpd : Inport  Port=4
  bol_flgShOffFlg : Inport  Port=5
  s16_nRefElecSpd : Inport  Port=6
  enm_stSysSt : Inport  Port=7
  u16_ampMaxVltgAmp : Inport  Port=8
  s16_uRefDaxVltgLim : Inport  Port=9
  s16_uRefQaxVltgLim : Inport  Port=10
  s16_pwrSplyElecPwr : Inport  Port=11
  Bus Creator1 : BusCreator  Inputs=11  OutDataTypeStr=Bus: BUS_AST_SLW_TASK_OUT  NonVirtualBus=on
      settings: InheritFromInputs=off
  busAST_SlwTaskOut : Outport
  wires:
  Bus Creator1/1 -> busAST_SlwTaskOut/1
  s16_iEstSplyCurr/1 -> Bus Creator1/1
  s16_ampActPhCurrAmp/1 -> Bus Creator1/2
  s16_trqRefTqLim/1 -> Bus Creator1/3
  s16_nRmpRefElecSpd/1 -> Bus Creator1/4
  bol_flgShOffFlg/1 -> Bus Creator1/5
  s16_nRefElecSpd/1 -> Bus Creator1/6
  enm_stSysSt/1 -> Bus Creator1/7
  u16_ampMaxVltgAmp/1 -> Bus Creator1/8
  s16_uRefDaxVltgLim/1 -> Bus Creator1/9
  s16_uRefQaxVltgLim/1 -> Bus Creator1/10
  s16_pwrSplyElecPwr/1 -> Bus Creator1/11

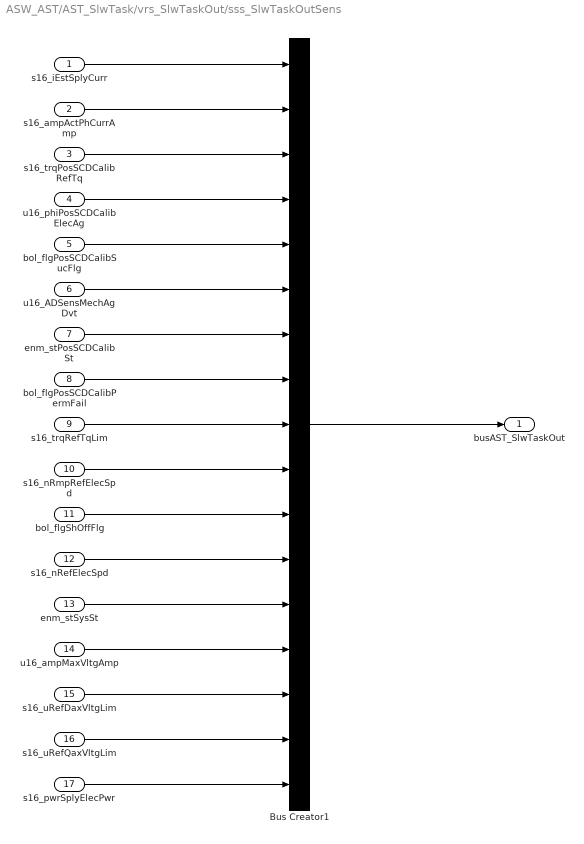
== system ASW_AST/AST_SlwTask/vrs_SlwTaskOut/sss_SlwTaskOutSens ==
  s16_iEstSplyCurr : Inport
  s16_ampActPhCurrAmp : Inport  Port=2
  s16_trqPosSCDCalibRefTq : Inport  Port=3
  u16_phiPosSCDCalibElecAg : Inport  Port=4
  bol_flgPosSCDCalibSucFlg : Inport  Port=5
  u16_ADSensMechAgDvt : Inport  Port=6
  enm_stPosSCDCalibSt : Inport  Port=7
  bol_flgPosSCDCalibPermFail : Inport  Port=8
  s16_trqRefTqLim : Inport  Port=9
  s16_nRmpRefElecSpd : Inport  Port=10
  bol_flgShOffFlg : Inport  Port=11
  s16_nRefElecSpd : Inport  Port=12
  enm_stSysSt : Inport  Port=13
  u16_ampMaxVltgAmp : Inport  Port=14
  s16_uRefDaxVltgLim : Inport  Port=15
  s16_uRefQaxVltgLim : Inport  Port=16
  s16_pwrSplyElecPwr : Inport  Port=17
  Bus Creator1 : BusCreator  Inputs=17  OutDataTypeStr=Bus: BUS_AST_SLW_TASK_OUT  NonVirtualBus=on
      settings: InheritFromInputs=off
  busAST_SlwTaskOut : Outport
  wires:
  s16_iEstSplyCurr/1 -> Bus Creator1/1
  s16_ampActPhCurrAmp/1 -> Bus Creator1/2
  s16_trqPosSCDCalibRefTq/1 -> Bus Creator1/3
  u16_phiPosSCDCalibElecAg/1 -> Bus Creator1/4
  bol_flgPosSCDCalibSucFlg/1 -> Bus Creator1/5
  u16_ADSensMechAgDvt/1 -> Bus Creator1/6
  enm_stPosSCDCalibSt/1 -> Bus Creator1/7
  bol_flgPosSCDCalibPermFail/1 -> Bus Creator1/8
  s16_trqRefTqLim/1 -> Bus Creator1/9
  s16_nRmpRefElecSpd/1 -> Bus Creator1/10
  bol_flgShOffFlg/1 -> Bus Creator1/11
  s16_nRefElecSpd/1 -> Bus Creator1/12
  enm_stSysSt/1 -> Bus Creator1/13
  Bus Creator1/1 -> busAST_SlwTaskOut/1
  u16_ampMaxVltgAmp/1 -> Bus Creator1/14
  s16_uRefDaxVltgLim/1 -> Bus Creator1/15
  s16_uRefQaxVltgLim/1 -> Bus Creator1/16
  s16_pwrSplyElecPwr/1 -> Bus Creator1/17
